simulink model "csc_cmg_meme_interface_hrn"  (R2014b)
settings: Solver=FixedStepDiscrete  StartTime=0.0  StopTime=1  FixedStep=1  RelTol=1e-3
values from neighbouring files (symbols this model uses):
  cam_cam1_lander_dcm = rot_angles_to_dcm( [cam_cam1_lander_rotz cam_cam1_lander_roty cam_cam1_lander_rotx] )    [csc_cam_camera_system_prep.m]
  cam_cam1_lander_quat = rot_angles_to_quat( [cam_cam1_lander_rotz cam_cam1_lander_roty cam_cam1_lander_rotx] )    [csc_cam_camera_system_prep.m]
undefined symbols (not defined in the file or in its folder): body_pos_eci, body_quat_eci, time
libraries: util_frame_rotation_lib x2, csc_cmg_camera_geometry_lib x1
settings Model: Creator=escrane  LastModifiedBy=mstewart
settings DebuggingCC: UnderspecifiedInitializationDetection=Classic  MergeDetectMultiDrivingBlocksExec=none  StateNameClashWarn=warning

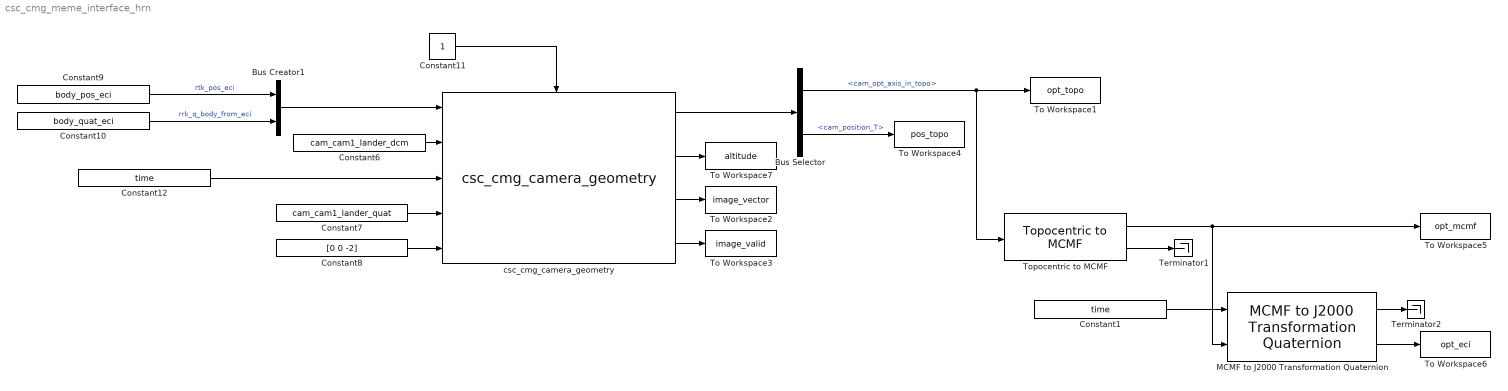
== system csc_cmg_meme_interface_hrn ==
  Bus Creator1 : BusCreator  Inputs=2
  Bus Selector : BusSelector  OutputSignals=cam_opt_axis_in_topo,cam_position_T
  Constant1 : Constant  Value=time
  Constant10 : Constant  Value=body_quat_eci
  Constant11 : Constant
  Constant12 : Constant  Value=time
  Constant6 : Constant  Value=cam_cam1_lander_dcm
  Constant7 : Constant  Value=cam_cam1_lander_quat
  Constant8 : Constant  Value=[0 0 -2]
  Constant9 : Constant  Value=body_pos_eci
  MCMF to J2000 Transformation Quaternion : util_frame_rotation_lib/MCMF to J2000  Transformation Quaternion
  Terminator1 : Terminator
  Terminator2 : Terminator
  To Workspace1 : ToWorkspace  VariableName=opt_topo  SaveFormat=Timeseries  SampleTime=-1
  To Workspace2 : ToWorkspace  VariableName=image_vector  SaveFormat=Timeseries  SampleTime=-1
  To Workspace3 : ToWorkspace  VariableName=image_valid  SaveFormat=Timeseries  SampleTime=-1
  To Workspace4 : ToWorkspace  VariableName=pos_topo  SaveFormat=Timeseries  SampleTime=-1
  To Workspace5 : ToWorkspace  VariableName=opt_mcmf  SaveFormat=Timeseries  SampleTime=-1
  To Workspace6 : ToWorkspace  VariableName=opt_eci  SaveFormat=Timeseries  SampleTime=-1
  To Workspace7 : ToWorkspace  VariableName=altitude  SaveFormat=Timeseries  SampleTime=-1
  Topocentric to MCMF : util_frame_rotation_lib/Topocentric to MCMF  SystemSampleTime=-1
  csc_cmg_camera_geometry : csc_cmg_camera_geometry_lib/csc_cmg_camera_geometry
  wires:
  Constant6/1 -> csc_cmg_camera_geometry/2
  Constant7/1 -> csc_cmg_camera_geometry/4
  Constant8/1 -> csc_cmg_camera_geometry/5
  Constant9/1 -> Bus Creator1/1  "rtk_pos_eci"
  Bus Creator1/1 -> csc_cmg_camera_geometry/1
  Constant10/1 -> Bus Creator1/2  "rrk_q_body_from_eci"
  Constant11/1 -> csc_cmg_camera_geometry/Enable
  Constant12/1 -> csc_cmg_camera_geometry/3
  csc_cmg_camera_geometry/1 -> Bus Selector/1
  Bus Selector/1 -> Topocentric to MCMF/1, To Workspace1/1  "<cam_opt_axis_in_topo>"
  Bus Selector/2 -> To Workspace4/1  "<cam_position_T>"
  Topocentric to MCMF/1 -> MCMF to J2000 Transformation Quaternion/2, To Workspace5/1
  Constant1/1 -> MCMF to J2000 Transformation Quaternion/1
  MCMF to J2000 Transformation Quaternion/2 -> To Workspace6/1
  Topocentric to MCMF/2 -> Terminator1/1
  MCMF to J2000 Transformation Quaternion/1 -> Terminator2/1
  csc_cmg_camera_geometry/4 -> To Workspace3/1
  csc_cmg_camera_geometry/3 -> To Workspace2/1
  csc_cmg_camera_geometry/2 -> To Workspace7/1
